simulink model "model_1"  (R2018a)
settings: Solver=VariableStepAuto  StartTime=0.0  StopTime=10  RelTol=1e-3
values from neighbouring files (symbols this model uses):
  a0 = 1    [anal_c_d.m]    (also in symulacyjne3B.m)
  a1 = 1    [anal_c_d.m]    (also in symulacyjne3B.m)
  b = 2    [anal_c_d.m]    (also in symulacyjne3B.m)
  t0 = 0    [anal_c_d.m]
  x0 = 2    [anal_c_d.m]
settings Model: Creator=johnb  LastModifiedBy=margr

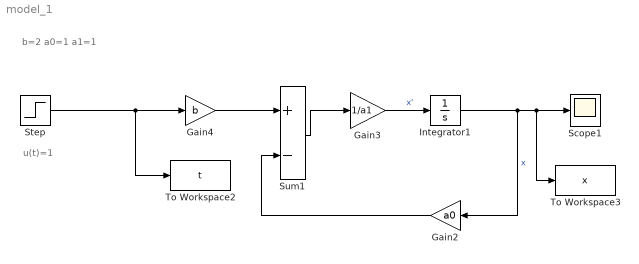
== system model_1 ==
  note: u(t)=1
  note: b=2
      | a0=1
      | a1=1
  Gain2 : Gain  Gain=a0
  Gain3 : Gain  Gain=1/a1
  Gain4 : Gain  Gain=b
  Integrator1 : Integrator  InitialCondition=x0
  Scope1 : Scope
  Step : Step  Time=t0  Before=x0  After=u  SampleTime=0
  Sum1 : Sum  Inputs=+-
  To Workspace2 : ToWorkspace  VariableName=t  SaveFormat=Timeseries  SampleTime=-1
  To Workspace3 : ToWorkspace  VariableName=x  SampleTime=-1
  wires:
  Integrator1/1 -> To Workspace3/1, Scope1/1, Gain2/1  "x"
  Gain3/1 -> Integrator1/1  "x'"
  Sum1/1 -> Gain3/1
  Gain2/1 -> Sum1/2
  Step/1 -> To Workspace2/1, Gain4/1
  Gain4/1 -> Sum1/1
